simulink model "bengji_fcn"  (R2021a)
settings: Solver=FixedStepAuto  StartTime=0.0  StopTime=50.0  FixedStep=0.1  RelTol=1e-3
model workspace (MAT data in the model file):
  times = 1
settings Model: Creator=86137  LastModifiedBy=86137

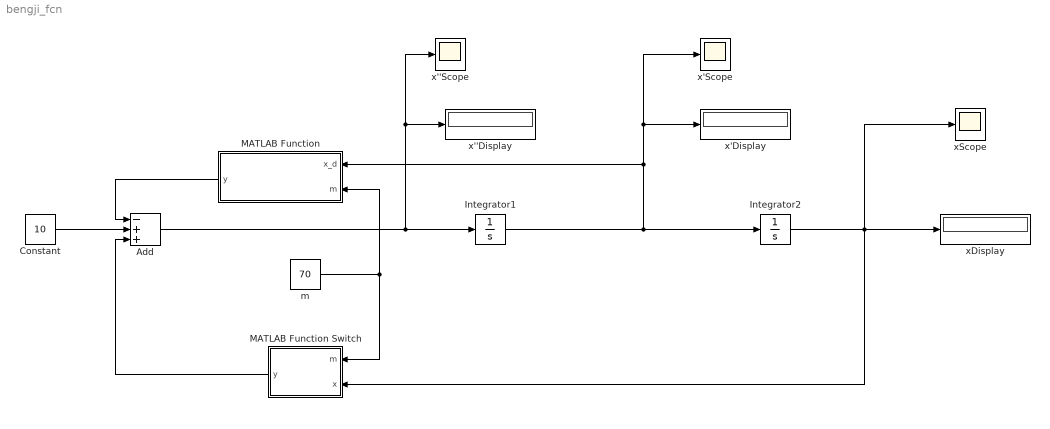
== system bengji_fcn ==
  Add : Sum  Inputs=-++
  Constant : Constant  Value=10
  Integrator1 : Integrator
  Integrator2 : Integrator  InitialCondition=-30
  MATLAB Function : MATLAB Function  TreatAsAtomicUnit=on
  MATLAB Function Switch : MATLAB Function  TreatAsAtomicUnit=on
  m : Constant  Value=70
  x''Display : Display
  x''Scope : Scope
  x'Display : Display
  x'Scope : Scope
  xDisplay : Display
  xScope : Scope
  wires:
  Constant/1 -> Add/2
  Add/1 -> x''Display/1, x''Scope/1, Integrator1/1
  Integrator1/1 -> x'Display/1, x'Scope/1, MATLAB Function/1(x_d), Integrator2/1
  Integrator2/1 -> MATLAB Function Switch/2(x), xScope/1, xDisplay/1
  MATLAB Function Switch/1(y) -> Add/3
  m/1 -> MATLAB Function Switch/1(m), MATLAB Function/2(m)
  MATLAB Function/1(y) -> Add/1

== matlab function bengji_fcn/MATLAB Function Switch ==
  data: m input; x input; y output
function y = fcn_switch(m,x)
if x>0
    b = -50*x;
else
    b = 0;
end
y = (b-x)/m;

== matlab function bengji_fcn/MATLAB Function ==
  data: x_d input; y output; m input
function y = fcn_abs_product(x_d,m)
a_x_d = abs(x_d);
y = a_x_d*x_d/m;
